simulink subsystem "uart_subsystem"  (R2025b)
settings: Solver=VariableStepAuto  StartTime=0.0  StopTime=10.0  RelTol=1e-3
libraries: c280xlib x2, svdutilitieslib x1
settings Model: Creator=orang  LastModifiedBy=erik

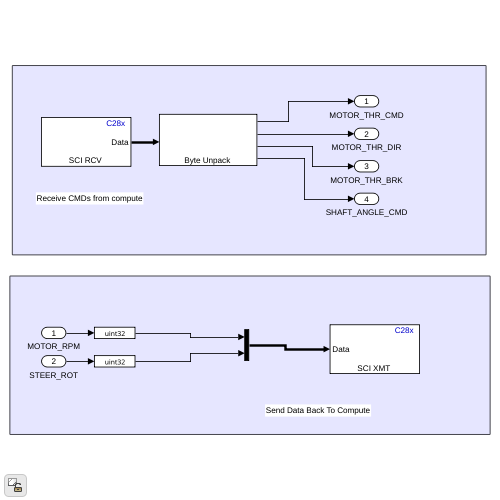
[thumbnail: Simulink's stored preview of the top-level diagram]
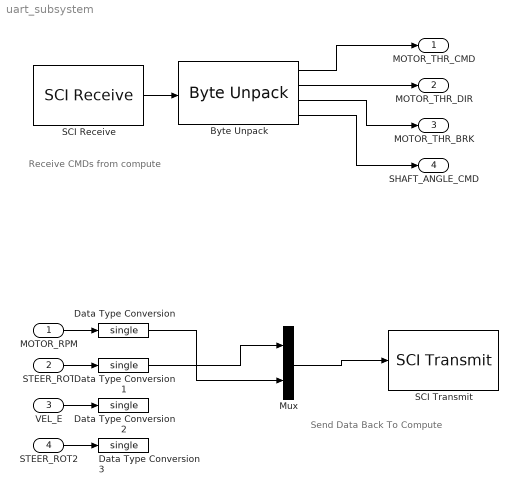
== system uart_subsystem ==
  note: Send Data Back To Compute
  note: Receive CMDs from compute
  MOTOR_RPM : Inport
  STEER_ROT : Inport  Port=2
  VEL_E : Inport  Port=3
  STEER_ROT2 : Inport  Port=4
  Byte Unpack : svdutilitieslib/Byte Unpack  dimensions={[1],[1],[1],[1]}  datatypes={'single','boolean','boolean','single'}  byteAlign=1  blockPlatform=tic2000
      settings: LibrarySourceBlock=c2000lib/Target Communication/Byte Unpack
  Data Type Conversion{,1..3} (4 alike) : DataTypeConversion  OutDataTypeStr=single  SaturateOnIntegerOverflow=off  RndMeth=Floor
  Mux : Mux  Inputs=2
  SCI Receive : c280xlib/SCI Receive  Priority=2  sciModule=A  dataHead=''  headerCheckMaxCount=16  dataTail=''  dataType=uint8  dataLenOptions=Length via dialog  dataDim=10  maxDataLength=1  initValue=0  errOption=Output the last received value  errValue=0  sampleTime=-1  blockingMode=off  timeOut=inf  outputStatus=off
      settings: LibrarySourceBlock=c2837xDlib/SCI Receive
  SCI Transmit : c280xlib/SCI Transmit  sciModule=A  dataHead=170  dataTail=85  frameSize=1  blockingMode=off  outputStatus=off
      settings: LibrarySourceBlock=c2837xDlib/SCI Transmit
  MOTOR_THR_CMD : Outport
  MOTOR_THR_DIR : Outport  Port=2
  MOTOR_THR_BRK : Outport  Port=3
  SHAFT_ANGLE_CMD : Outport  Port=4
  wires:
  Byte Unpack/2 -> MOTOR_THR_DIR/1
  Byte Unpack/3 -> MOTOR_THR_BRK/1
  Byte Unpack/4 -> SHAFT_ANGLE_CMD/1
  SCI Receive/1 -> Byte Unpack/1
  Byte Unpack/1 -> MOTOR_THR_CMD/1
  STEER_ROT/1 -> Data Type Conversion1/1
  MOTOR_RPM/1 -> Data Type Conversion/1
  Mux/1 -> SCI Transmit/1
  VEL_E/1 -> Data Type Conversion2/1
  STEER_ROT2/1 -> Data Type Conversion3/1
  Data Type Conversion/1 -> Mux/2
  Data Type Conversion1/1 -> Mux/1
